simulink model "adc1x12_10g"  (R2019a)
settings: Solver=VariableStepAuto  StartTime=0.0  StopTime=10.0  RelTol=1e-3
libraries: xbsIndex_r4 x32
settings Model: Creator=qwerty40  LastModifiedBy=jkocz
settings DataIOCC: ReturnWorkspaceOutputs=off
settings DebuggingCC: ArithmeticOperatorsInVariantConditions=warning
settings SFSimCC: SimUseLocalCustomCode=off
settings RTWCC: RTWUseLocalCustomCode=off
settings CodeAppCC: StateflowObjectComments=on

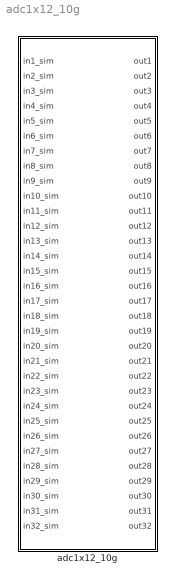
== system adc1x12_10g ==
  adc1x12_10g : Subsystem  Tag=xps:snap_adc  mask(adc1x12_10g){}
      mask help: Interface to the 1 adc chip on the HTG FMC board. Please see Help for instructions on parameter settings
      mask init:
      | adc1x12_10g_mask(gcb);
      mask Help:
      | This is the CASPER "yellow block" for the ADCs on the HG FMC board.
      | Each ADC chip accepts one input.
      | 
      | Maximum sample rate f (Mega samples per second)
      | 
      | Number of inputs         1
      | Resolution 12 bits        f=10000

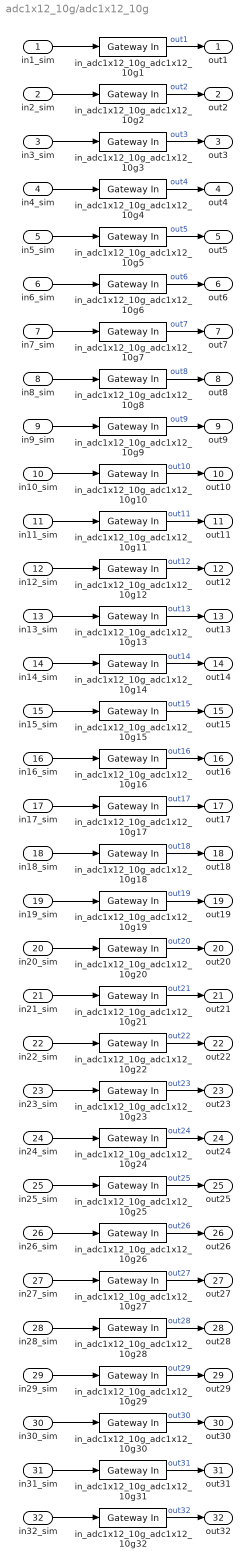
== system adc1x12_10g/adc1x12_10g ==
  in1_sim : Inport
  in2_sim : Inport  Port=2
  in3_sim : Inport  Port=3
  in4_sim : Inport  Port=4
  in5_sim : Inport  Port=5
  in6_sim : Inport  Port=6
  in7_sim : Inport  Port=7
  in8_sim : Inport  Port=8
  in9_sim : Inport  Port=9
  in10_sim : Inport  Port=10
  in11_sim : Inport  Port=11
  in12_sim : Inport  Port=12
  in13_sim : Inport  Port=13
  in14_sim : Inport  Port=14
  in15_sim : Inport  Port=15
  in16_sim : Inport  Port=16
  in17_sim : Inport  Port=17
  in18_sim : Inport  Port=18
  in19_sim : Inport  Port=19
  in20_sim : Inport  Port=20
  in21_sim : Inport  Port=21
  in22_sim : Inport  Port=22
  in23_sim : Inport  Port=23
  in24_sim : Inport  Port=24
  in25_sim : Inport  Port=25
  in26_sim : Inport  Port=26
  in27_sim : Inport  Port=27
  in28_sim : Inport  Port=28
  in29_sim : Inport  Port=29
  in30_sim : Inport  Port=30
  in31_sim : Inport  Port=31
  in32_sim : Inport  Port=32
  in_adc1x12_10g_adc1x12_10g{1..32} (32 alike) : xbsIndex_r4/Gateway In  gui_display_data_type=Fixed-point  arith_type="Signed  (2's comp)"  n_bits=12  bin_pt=11  preci_type=Single  exp_width=8  frac_width=24  rows=1  columns=1  quantization="Round  (unbiased: +/- Inf)"  overflow=Saturate  period=1  UseAsADC=off  ADCChannel='1'  interface=None  automatic_assignment=on  address_offset=hex2dec('00')  intf_name=''  intf_description=''  default_value=0  timing_constraint=None  locs_specified=off  LOCs={}  io_standard={}  inherit_from_input=off  hdl_port=on  dbl_ovrd=off  block_type=gatewayin
  out1 : Outport
  out2 : Outport  Port=2
  out3 : Outport  Port=3
  out4 : Outport  Port=4
  out5 : Outport  Port=5
  out6 : Outport  Port=6
  out7 : Outport  Port=7
  out8 : Outport  Port=8
  out9 : Outport  Port=9
  out10 : Outport  Port=10
  out11 : Outport  Port=11
  out12 : Outport  Port=12
  out13 : Outport  Port=13
  out14 : Outport  Port=14
  out15 : Outport  Port=15
  out16 : Outport  Port=16
  out17 : Outport  Port=17
  out18 : Outport  Port=18
  out19 : Outport  Port=19
  out20 : Outport  Port=20
  out21 : Outport  Port=21
  out22 : Outport  Port=22
  out23 : Outport  Port=23
  out24 : Outport  Port=24
  out25 : Outport  Port=25
  out26 : Outport  Port=26
  out27 : Outport  Port=27
  out28 : Outport  Port=28
  out29 : Outport  Port=29
  out30 : Outport  Port=30
  out31 : Outport  Port=31
  out32 : Outport  Port=32
  wires:
  in1_sim/1 -> in_adc1x12_10g_adc1x12_10g1/1
  in_adc1x12_10g_adc1x12_10g1/1 -> out1/1  "out1"
  in2_sim/1 -> in_adc1x12_10g_adc1x12_10g2/1
  in_adc1x12_10g_adc1x12_10g2/1 -> out2/1  "out2"
  in3_sim/1 -> in_adc1x12_10g_adc1x12_10g3/1
  in_adc1x12_10g_adc1x12_10g3/1 -> out3/1  "out3"
  in4_sim/1 -> in_adc1x12_10g_adc1x12_10g4/1
  in_adc1x12_10g_adc1x12_10g4/1 -> out4/1  "out4"
  in5_sim/1 -> in_adc1x12_10g_adc1x12_10g5/1
  in_adc1x12_10g_adc1x12_10g5/1 -> out5/1  "out5"
  in6_sim/1 -> in_adc1x12_10g_adc1x12_10g6/1
  in_adc1x12_10g_adc1x12_10g6/1 -> out6/1  "out6"
  in7_sim/1 -> in_adc1x12_10g_adc1x12_10g7/1
  in_adc1x12_10g_adc1x12_10g7/1 -> out7/1  "out7"
  in8_sim/1 -> in_adc1x12_10g_adc1x12_10g8/1
  in_adc1x12_10g_adc1x12_10g8/1 -> out8/1  "out8"
  in9_sim/1 -> in_adc1x12_10g_adc1x12_10g9/1
  in_adc1x12_10g_adc1x12_10g9/1 -> out9/1  "out9"
  in10_sim/1 -> in_adc1x12_10g_adc1x12_10g10/1
  in_adc1x12_10g_adc1x12_10g10/1 -> out10/1  "out10"
  in11_sim/1 -> in_adc1x12_10g_adc1x12_10g11/1
  in_adc1x12_10g_adc1x12_10g11/1 -> out11/1  "out11"
  in12_sim/1 -> in_adc1x12_10g_adc1x12_10g12/1
  in_adc1x12_10g_adc1x12_10g12/1 -> out12/1  "out12"
  in13_sim/1 -> in_adc1x12_10g_adc1x12_10g13/1
  in_adc1x12_10g_adc1x12_10g13/1 -> out13/1  "out13"
  in14_sim/1 -> in_adc1x12_10g_adc1x12_10g14/1
  in_adc1x12_10g_adc1x12_10g14/1 -> out14/1  "out14"
  in15_sim/1 -> in_adc1x12_10g_adc1x12_10g15/1
  in_adc1x12_10g_adc1x12_10g15/1 -> out15/1  "out15"
  in16_sim/1 -> in_adc1x12_10g_adc1x12_10g16/1
  in_adc1x12_10g_adc1x12_10g16/1 -> out16/1  "out16"
  in17_sim/1 -> in_adc1x12_10g_adc1x12_10g17/1
  in_adc1x12_10g_adc1x12_10g17/1 -> out17/1  "out17"
  in18_sim/1 -> in_adc1x12_10g_adc1x12_10g18/1
  in_adc1x12_10g_adc1x12_10g18/1 -> out18/1  "out18"
  in19_sim/1 -> in_adc1x12_10g_adc1x12_10g19/1
  in_adc1x12_10g_adc1x12_10g19/1 -> out19/1  "out19"
  in20_sim/1 -> in_adc1x12_10g_adc1x12_10g20/1
  in_adc1x12_10g_adc1x12_10g20/1 -> out20/1  "out20"
  in21_sim/1 -> in_adc1x12_10g_adc1x12_10g21/1
  in_adc1x12_10g_adc1x12_10g21/1 -> out21/1  "out21"
  in22_sim/1 -> in_adc1x12_10g_adc1x12_10g22/1
  in_adc1x12_10g_adc1x12_10g22/1 -> out22/1  "out22"
  in23_sim/1 -> in_adc1x12_10g_adc1x12_10g23/1
  in_adc1x12_10g_adc1x12_10g23/1 -> out23/1  "out23"
  in24_sim/1 -> in_adc1x12_10g_adc1x12_10g24/1
  in_adc1x12_10g_adc1x12_10g24/1 -> out24/1  "out24"
  in25_sim/1 -> in_adc1x12_10g_adc1x12_10g25/1
  in_adc1x12_10g_adc1x12_10g25/1 -> out25/1  "out25"
  in26_sim/1 -> in_adc1x12_10g_adc1x12_10g26/1
  in_adc1x12_10g_adc1x12_10g26/1 -> out26/1  "out26"
  in27_sim/1 -> in_adc1x12_10g_adc1x12_10g27/1
  in_adc1x12_10g_adc1x12_10g27/1 -> out27/1  "out27"
  in28_sim/1 -> in_adc1x12_10g_adc1x12_10g28/1
  in_adc1x12_10g_adc1x12_10g28/1 -> out28/1  "out28"
  in29_sim/1 -> in_adc1x12_10g_adc1x12_10g29/1
  in_adc1x12_10g_adc1x12_10g29/1 -> out29/1  "out29"
  in30_sim/1 -> in_adc1x12_10g_adc1x12_10g30/1
  in_adc1x12_10g_adc1x12_10g30/1 -> out30/1  "out30"
  in31_sim/1 -> in_adc1x12_10g_adc1x12_10g31/1
  in_adc1x12_10g_adc1x12_10g31/1 -> out31/1  "out31"
  in32_sim/1 -> in_adc1x12_10g_adc1x12_10g32/1
  in_adc1x12_10g_adc1x12_10g32/1 -> out32/1  "out32"
